simulink model "sdbe_8pac_11"  (R2012b)
settings: Solver=VariableStepDiscrete  SolverMode=SingleTasking  StartTime=0.0  StopTime=10000  RelTol=1e-3
PreLoadFcn:
  | counter_vals
undefined symbols (not defined in the file or in its folder): sfp
libraries: xbsIndex_r4 x9355, casper_library_misc x39, casper_library_delays x27, dspsigops x16, xps_library x10, r2dbe_vdif_lib x4, r2dbe_adc_lib x3, simulink x1
(part 1 of 79)
settings Model: Creator=lvertats  LastModifiedBy=ayoung
settings OptimizationCC: InlineParams=on

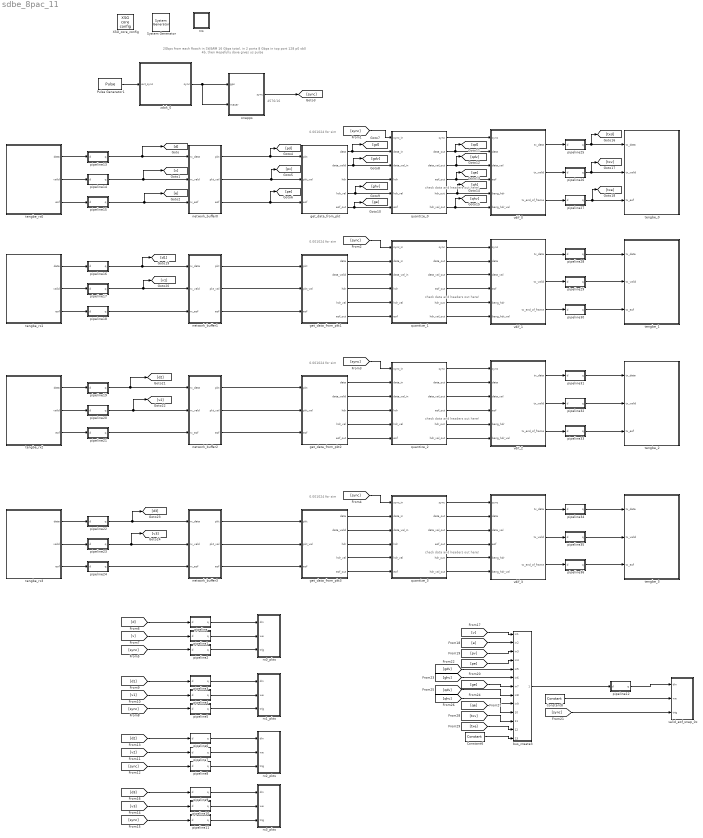
== system sdbe_8pac_11 ==
  note: 0.001024 for sim
  note: 4576/16
  note: check data and headers out here!
  note: 2Gbps from each Roach in SWARM
      | 16 Gbps total, in 2 ports
      | 8 Gbps in top port
      | 128 p0 sb0 4b, then
      |
      | Hopefully dave gives us pulse
  note: 0.001024 for sim
  note: check data and headers out here!
  note: 0.001024 for sim
  note: check data and headers out here!
  note: 0.001024 for sim
  note: check data and headers out here!
  " System Generator" : xbsIndex_r4/ System Generator  Tag=genX  xilinxfamily=virtex6  part=xc6vsx475t  speed=-1  package=ff1759  synthesis_tool=XST  clock_wrapper=Clock Enables  directory=./sdbe_8pac_11/sysgen  proj_type=Project Navigator  Synth_file=XST Defaults  Impl_file=ISE Defaults  testbench=off  simulink_period=1  sysclk_period=3.4965  dcm_input_clock_period=100  incr_netlist=off  trim_vbits=Everywhere in SubSystem  dbl_ovrd=According to Block Masks  core_generation=According to Block Masks  run_coregen=off  deprecated_control=off  eval_field=0  block_type=sysgen
  Constant6 : xbsIndex_r4/Constant  const=0  gui_display_data_type=Fixed-point  arith_type=Unsigned  n_bits=4  bin_pt=0  preci_type=Single  exp_width=8  frac_width=24  explicit_period=on  period=1  equ=P=C  opselect=C  inp2=PCIN>>17  opr=+  inp1=P  carry=CIN  dbl_ovrd=off  block_type=constant
  Constant8 : xbsIndex_r4/Constant  const=1  gui_display_data_type=Boolean  arith_type=Boolean  n_bits=31  bin_pt=0  preci_type=Single  exp_width=8  frac_width=24  explicit_period=on  period=1  equ=P=C  opselect=C  inp2=PCIN>>17  opr=+  inp1=P  carry=CIN  dbl_ovrd=off  block_type=constant
  Pulse Generator1 : DiscretePulseGenerator  Period=1024  PhaseDelay=57
  XSG_core_config : xps_library/XSG core config  Tag=xps:xsg  hw_sys=ROACH2:sx475t  clk_src=adc0_clk  ROACH_clk_src=sys_clk  ROACH2_clk_src=adc0_clk  MKDIG_clk_src=sys_clk  clk_rate=4576/16  sample_period=1  synthesis_tool=XST
  bus_create3 : Subsystem  AncestorBlock=casper_library_flow_control/bus_create  mask(bus_create){inputNum=13}
      mask prompts: inputNum "Number of inputs:"
      mask init:
      | bus_create_init(gcb,...
      |     'inputNum', inputNum);
  get_data_from_pkt : Subsystem
  get_data_from_pkt1 : Subsystem
  get_data_from_pkt2 : Subsystem
  get_data_from_pkt3 : Subsystem
  network_buffer0 : Subsystem  mask{pipe_delay=4}
      mask prompts: pipe_delay "Pipeline delay:"
      mask init:
      | set_param([gcb '/pipe_din'],'latency',pipe_delay)
      | set_param([gcb '/pipe_we'],'latency',pipe_delay)
      | set_param([gcb '/pipe_re'],'latency',pipe_delay)
      | set_param([gcb '/pipe_eof'],'latency',pipe_delay)
  network_buffer1 : Subsystem  mask{pipe_delay=4}
      mask prompts: pipe_delay "Pipeline delay:"
      mask init:
      | set_param([gcb '/pipe_din'],'latency',pipe_delay)
      | set_param([gcb '/pipe_we'],'latency',pipe_delay)
      | set_param([gcb '/pipe_re'],'latency',pipe_delay)
      | set_param([gcb '/pipe_eof'],'latency',pipe_delay)
  network_buffer2 : Subsystem  mask{pipe_delay=4}
      mask prompts: pipe_delay "Pipeline delay:"
      mask init:
      | set_param([gcb '/pipe_din'],'latency',pipe_delay)
      | set_param([gcb '/pipe_we'],'latency',pipe_delay)
      | set_param([gcb '/pipe_re'],'latency',pipe_delay)
      | set_param([gcb '/pipe_eof'],'latency',pipe_delay)
  network_buffer3 : Subsystem  mask{pipe_delay=4}
      mask prompts: pipe_delay "Pipeline delay:"
      mask init:
      | set_param([gcb '/pipe_din'],'latency',pipe_delay)
      | set_param([gcb '/pipe_we'],'latency',pipe_delay)
      | set_param([gcb '/pipe_re'],'latency',pipe_delay)
      | set_param([gcb '/pipe_eof'],'latency',pipe_delay)
  onepps : Subsystem  AncestorBlock=r2dbe_adc_lib/onepps  mask(r2dbe_onepps){clk_rate=4576/16}
      mask prompts: clk_rate "FPGA clock rate (MHz):"
      mask help: Sub-system for 1pps parameters of the R2DBE.
  pipeline : Subsystem  AncestorBlock=casper_library_delays/pipeline  mask(pipeline){latency=16}
      mask help:
      | An explicitly laid-out delay line to avoid mapping to SRL16s
      | for use in pipelining to help achieve timing closure.
      mask init:
      | pipeline_init(gcb,'latency',latency);
      settings: AttributesFormatString=Latency = %<latency>
      mask Display:
      | port_label('input', 1, 'd');
      | port_label('output', 1, 'q');
      | disp(['Z^-', num2str(latency)]);
  pipeline1 : Subsystem  AncestorBlock=casper_library_delays/pipeline  mask(pipeline){latency=16}
      mask help:
      | An explicitly laid-out delay line to avoid mapping to SRL16s
      | for use in pipelining to help achieve timing closure.
      mask init:
      | pipeline_init(gcb,'latency',latency);
      settings: AttributesFormatString=Latency = %<latency>
      mask Display:
      | port_label('input', 1, 'd');
      | port_label('output', 1, 'q');
      | disp(['Z^-', num2str(latency)]);
  pipeline10 : Subsystem  AncestorBlock=casper_library_delays/pipeline  mask(pipeline){latency=16}
      mask help:
      | An explicitly laid-out delay line to avoid mapping to SRL16s
      | for use in pipelining to help achieve timing closure.
      mask init:
      | pipeline_init(gcb,'latency',latency);
      settings: AttributesFormatString=Latency = %<latency>
      mask Display:
      | port_label('input', 1, 'd');
      | port_label('output', 1, 'q');
      | disp(['Z^-', num2str(latency)]);
  pipeline11 : Subsystem  AncestorBlock=casper_library_delays/pipeline  mask(pipeline){latency=16}
      mask help:
      | An explicitly laid-out delay line to avoid mapping to SRL16s
      | for use in pipelining to help achieve timing closure.
      mask init:
      | pipeline_init(gcb,'latency',latency);
      settings: AttributesFormatString=Latency = %<latency>
      mask Display:
      | port_label('input', 1, 'd');
      | port_label('output', 1, 'q');
      | disp(['Z^-', num2str(latency)]);
  pipeline12 : Subsystem  AncestorBlock=casper_library_delays/pipeline  mask(pipeline){latency=16}
      mask help:
      | An explicitly laid-out delay line to avoid mapping to SRL16s
      | for use in pipelining to help achieve timing closure.
      mask init:
      | pipeline_init(gcb,'latency',latency);
      settings: AttributesFormatString=Latency = %<latency>
      mask Display:
      | port_label('input', 1, 'd');
      | port_label('output', 1, 'q');
      | disp(['Z^-', num2str(latency)]);
  pipeline13 : Subsystem  AncestorBlock=casper_library_delays/pipeline  mask(pipeline){latency=4}
      mask help:
      | An explicitly laid-out delay line to avoid mapping to SRL16s
      | for use in pipelining to help achieve timing closure.
      mask init:
      | pipeline_init(gcb,'latency',latency);
      settings: AttributesFormatString=Latency = %<latency>
      mask Display:
      | port_label('input', 1, 'd');
      | port_label('output', 1, 'q');
      | disp(['Z^-', num2str(latency)]);
  pipeline14 : Subsystem  AncestorBlock=casper_library_delays/pipeline  mask(pipeline){latency=4}
      mask help:
      | An explicitly laid-out delay line to avoid mapping to SRL16s
      | for use in pipelining to help achieve timing closure.
      mask init:
      | pipeline_init(gcb,'latency',latency);
      settings: AttributesFormatString=Latency = %<latency>
      mask Display:
      | port_label('input', 1, 'd');
      | port_label('output', 1, 'q');
      | disp(['Z^-', num2str(latency)]);
  pipeline15 : Subsystem  AncestorBlock=casper_library_delays/pipeline  mask(pipeline){latency=4}
      mask help:
      | An explicitly laid-out delay line to avoid mapping to SRL16s
      | for use in pipelining to help achieve timing closure.
      mask init:
      | pipeline_init(gcb,'latency',latency);
      settings: AttributesFormatString=Latency = %<latency>
      mask Display:
      | port_label('input', 1, 'd');
      | port_label('output', 1, 'q');
      | disp(['Z^-', num2str(latency)]);
  pipeline16 : Subsystem  AncestorBlock=casper_library_delays/pipeline  mask(pipeline){latency=4}
      mask help:
      | An explicitly laid-out delay line to avoid mapping to SRL16s
      | for use in pipelining to help achieve timing closure.
      mask init:
      | pipeline_init(gcb,'latency',latency);
      settings: AttributesFormatString=Latency = %<latency>
      mask Display:
      | port_label('input', 1, 'd');
      | port_label('output', 1, 'q');
      | disp(['Z^-', num2str(latency)]);
  pipeline17 : Subsystem  AncestorBlock=casper_library_delays/pipeline  mask(pipeline){latency=4}
      mask help:
      | An explicitly laid-out delay line to avoid mapping to SRL16s
      | for use in pipelining to help achieve timing closure.
      mask init:
      | pipeline_init(gcb,'latency',latency);
      settings: AttributesFormatString=Latency = %<latency>
      mask Display:
      | port_label('input', 1, 'd');
      | port_label('output', 1, 'q');
      | disp(['Z^-', num2str(latency)]);
  pipeline18 : Subsystem  AncestorBlock=casper_library_delays/pipeline  mask(pipeline){latency=4}
      mask help:
      | An explicitly laid-out delay line to avoid mapping to SRL16s
      | for use in pipelining to help achieve timing closure.
      mask init:
      | pipeline_init(gcb,'latency',latency);
      settings: AttributesFormatString=Latency = %<latency>
      mask Display:
      | port_label('input', 1, 'd');
      | port_label('output', 1, 'q');
      | disp(['Z^-', num2str(latency)]);
  pipeline19 : Subsystem  AncestorBlock=casper_library_delays/pipeline  mask(pipeline){latency=4}
      mask help:
      | An explicitly laid-out delay line to avoid mapping to SRL16s
      | for use in pipelining to help achieve timing closure.
      mask init:
      | pipeline_init(gcb,'latency',latency);
      settings: AttributesFormatString=Latency = %<latency>
      mask Display:
      | port_label('input', 1, 'd');
      | port_label('output', 1, 'q');
      | disp(['Z^-', num2str(latency)]);
  pipeline2 : Subsystem  AncestorBlock=casper_library_delays/pipeline  mask(pipeline){latency=16}
      mask help:
      | An explicitly laid-out delay line to avoid mapping to SRL16s
      | for use in pipelining to help achieve timing closure.
      mask init:
      | pipeline_init(gcb,'latency',latency);
      settings: AttributesFormatString=Latency = %<latency>
      mask Display:
      | port_label('input', 1, 'd');
      | port_label('output', 1, 'q');
      | disp(['Z^-', num2str(latency)]);
  pipeline20 : Subsystem  AncestorBlock=casper_library_delays/pipeline  mask(pipeline){latency=4}
      mask help:
      | An explicitly laid-out delay line to avoid mapping to SRL16s
      | for use in pipelining to help achieve timing closure.
      mask init:
      | pipeline_init(gcb,'latency',latency);
      settings: AttributesFormatString=Latency = %<latency>
      mask Display:
      | port_label('input', 1, 'd');
      | port_label('output', 1, 'q');
      | disp(['Z^-', num2str(latency)]);
  pipeline21 : Subsystem  AncestorBlock=casper_library_delays/pipeline  mask(pipeline){latency=4}
      mask help:
      | An explicitly laid-out delay line to avoid mapping to SRL16s
      | for use in pipelining to help achieve timing closure.
      mask init:
      | pipeline_init(gcb,'latency',latency);
      settings: AttributesFormatString=Latency = %<latency>
      mask Display:
      | port_label('input', 1, 'd');
      | port_label('output', 1, 'q');
      | disp(['Z^-', num2str(latency)]);
  pipeline22 : Subsystem  AncestorBlock=casper_library_delays/pipeline  mask(pipeline){latency=4}
      mask help:
      | An explicitly laid-out delay line to avoid mapping to SRL16s
      | for use in pipelining to help achieve timing closure.
      mask init:
      | pipeline_init(gcb,'latency',latency);
      settings: AttributesFormatString=Latency = %<latency>
      mask Display:
      | port_label('input', 1, 'd');
      | port_label('output', 1, 'q');
      | disp(['Z^-', num2str(latency)]);
  pipeline23 : Subsystem  AncestorBlock=casper_library_delays/pipeline  mask(pipeline){latency=4}
      mask help:
      | An explicitly laid-out delay line to avoid mapping to SRL16s
      | for use in pipelining to help achieve timing closure.
      mask init:
      | pipeline_init(gcb,'latency',latency);
      settings: AttributesFormatString=Latency = %<latency>
      mask Display:
      | port_label('input', 1, 'd');
      | port_label('output', 1, 'q');
      | disp(['Z^-', num2str(latency)]);
  pipeline24 : Subsystem  AncestorBlock=casper_library_delays/pipeline  mask(pipeline){latency=4}
      mask help:
      | An explicitly laid-out delay line to avoid mapping to SRL16s
      | for use in pipelining to help achieve timing closure.
      mask init:
      | pipeline_init(gcb,'latency',latency);
      settings: AttributesFormatString=Latency = %<latency>
      mask Display:
      | port_label('input', 1, 'd');
      | port_label('output', 1, 'q');
      | disp(['Z^-', num2str(latency)]);
  pipeline25 : Subsystem  AncestorBlock=casper_library_delays/pipeline  mask(pipeline){latency=4}
      mask help:
      | An explicitly laid-out delay line to avoid mapping to SRL16s
      | for use in pipelining to help achieve timing closure.
      mask init:
      | pipeline_init(gcb,'latency',latency);
      settings: AttributesFormatString=Latency = %<latency>
      mask Display:
      | port_label('input', 1, 'd');
      | port_label('output', 1, 'q');
      | disp(['Z^-', num2str(latency)]);
  pipeline26 : Subsystem  AncestorBlock=casper_library_delays/pipeline  mask(pipeline){latency=4}
      mask help:
      | An explicitly laid-out delay line to avoid mapping to SRL16s
      | for use in pipelining to help achieve timing closure.
      mask init:
      | pipeline_init(gcb,'latency',latency);
      settings: AttributesFormatString=Latency = %<latency>
      mask Display:
      | port_label('input', 1, 'd');
      | port_label('output', 1, 'q');
      | disp(['Z^-', num2str(latency)]);
  pipeline27 : Subsystem  AncestorBlock=casper_library_delays/pipeline  mask(pipeline){latency=4}
      mask help:
      | An explicitly laid-out delay line to avoid mapping to SRL16s
      | for use in pipelining to help achieve timing closure.
      mask init:
      | pipeline_init(gcb,'latency',latency);
      settings: AttributesFormatString=Latency = %<latency>
      mask Display:
      | port_label('input', 1, 'd');
      | port_label('output', 1, 'q');
      | disp(['Z^-', num2str(latency)]);
  pipeline28 : Subsystem  AncestorBlock=casper_library_delays/pipeline  mask(pipeline){latency=4}
      mask help:
      | An explicitly laid-out delay line to avoid mapping to SRL16s
      | for use in pipelining to help achieve timing closure.
      mask init:
      | pipeline_init(gcb,'latency',latency);
      settings: AttributesFormatString=Latency = %<latency>
      mask Display:
      | port_label('input', 1, 'd');
      | port_label('output', 1, 'q');
      | disp(['Z^-', num2str(latency)]);
  pipeline29 : Subsystem  AncestorBlock=casper_library_delays/pipeline  mask(pipeline){latency=4}
      mask help:
      | An explicitly laid-out delay line to avoid mapping to SRL16s
      | for use in pipelining to help achieve timing closure.
      mask init:
      | pipeline_init(gcb,'latency',latency);
      settings: AttributesFormatString=Latency = %<latency>
      mask Display:
      | port_label('input', 1, 'd');
      | port_label('output', 1, 'q');
      | disp(['Z^-', num2str(latency)]);
  pipeline3 : Subsystem  AncestorBlock=casper_library_delays/pipeline  mask(pipeline){latency=16}
      mask help:
      | An explicitly laid-out delay line to avoid mapping to SRL16s
      | for use in pipelining to help achieve timing closure.
      mask init:
      | pipeline_init(gcb,'latency',latency);
      settings: AttributesFormatString=Latency = %<latency>
      mask Display:
      | port_label('input', 1, 'd');
      | port_label('output', 1, 'q');
      | disp(['Z^-', num2str(latency)]);
  pipeline30 : Subsystem  AncestorBlock=casper_library_delays/pipeline  mask(pipeline){latency=4}
      mask help:
      | An explicitly laid-out delay line to avoid mapping to SRL16s
      | for use in pipelining to help achieve timing closure.
      mask init:
      | pipeline_init(gcb,'latency',latency);
      settings: AttributesFormatString=Latency = %<latency>
      mask Display:
      | port_label('input', 1, 'd');
      | port_label('output', 1, 'q');
      | disp(['Z^-', num2str(latency)]);
  pipeline31 : Subsystem  AncestorBlock=casper_library_delays/pipeline  mask(pipeline){latency=4}
      mask help:
      | An explicitly laid-out delay line to avoid mapping to SRL16s
      | for use in pipelining to help achieve timing closure.
      mask init:
      | pipeline_init(gcb,'latency',latency);
      settings: AttributesFormatString=Latency = %<latency>
      mask Display:
      | port_label('input', 1, 'd');
      | port_label('output', 1, 'q');
      | disp(['Z^-', num2str(latency)]);
  pipeline32 : Subsystem  AncestorBlock=casper_library_delays/pipeline  mask(pipeline){latency=4}
      mask help:
      | An explicitly laid-out delay line to avoid mapping to SRL16s
      | for use in pipelining to help achieve timing closure.
      mask init:
      | pipeline_init(gcb,'latency',latency);
      settings: AttributesFormatString=Latency = %<latency>
      mask Display:
      | port_label('input', 1, 'd');
      | port_label('output', 1, 'q');
      | disp(['Z^-', num2str(latency)]);
  pipeline33 : Subsystem  AncestorBlock=casper_library_delays/pipeline  mask(pipeline){latency=4}
      mask help:
      | An explicitly laid-out delay line to avoid mapping to SRL16s
      | for use in pipelining to help achieve timing closure.
      mask init:
      | pipeline_init(gcb,'latency',latency);
      settings: AttributesFormatString=Latency = %<latency>
      mask Display:
      | port_label('input', 1, 'd');
      | port_label('output', 1, 'q');
      | disp(['Z^-', num2str(latency)]);
  pipeline34 : Subsystem  AncestorBlock=casper_library_delays/pipeline  mask(pipeline){latency=4}
      mask help:
      | An explicitly laid-out delay line to avoid mapping to SRL16s
      | for use in pipelining to help achieve timing closure.
      mask init:
      | pipeline_init(gcb,'latency',latency);
      settings: AttributesFormatString=Latency = %<latency>
      mask Display:
      | port_label('input', 1, 'd');
      | port_label('output', 1, 'q');
      | disp(['Z^-', num2str(latency)]);
  pipeline35 : Subsystem  AncestorBlock=casper_library_delays/pipeline  mask(pipeline){latency=4}
      mask help:
      | An explicitly laid-out delay line to avoid mapping to SRL16s
      | for use in pipelining to help achieve timing closure.
      mask init:
      | pipeline_init(gcb,'latency',latency);
      settings: AttributesFormatString=Latency = %<latency>
      mask Display:
      | port_label('input', 1, 'd');
      | port_label('output', 1, 'q');
      | disp(['Z^-', num2str(latency)]);
  pipeline36 : Subsystem  AncestorBlock=casper_library_delays/pipeline  mask(pipeline){latency=4}
      mask help:
      | An explicitly laid-out delay line to avoid mapping to SRL16s
      | for use in pipelining to help achieve timing closure.
      mask init:
      | pipeline_init(gcb,'latency',latency);
      settings: AttributesFormatString=Latency = %<latency>
      mask Display:
      | port_label('input', 1, 'd');
      | port_label('output', 1, 'q');
      | disp(['Z^-', num2str(latency)]);
  pipeline4 : Subsystem  AncestorBlock=casper_library_delays/pipeline  mask(pipeline){latency=16}
      mask help:
      | An explicitly laid-out delay line to avoid mapping to SRL16s
      | for use in pipelining to help achieve timing closure.
      mask init:
      | pipeline_init(gcb,'latency',latency);
      settings: AttributesFormatString=Latency = %<latency>
      mask Display:
      | port_label('input', 1, 'd');
      | port_label('output', 1, 'q');
      | disp(['Z^-', num2str(latency)]);
  pipeline5 : Subsystem  AncestorBlock=casper_library_delays/pipeline  mask(pipeline){latency=16}
      mask help:
      | An explicitly laid-out delay line to avoid mapping to SRL16s
      | for use in pipelining to help achieve timing closure.
      mask init:
      | pipeline_init(gcb,'latency',latency);
      settings: AttributesFormatString=Latency = %<latency>
      mask Display:
      | port_label('input', 1, 'd');
      | port_label('output', 1, 'q');
      | disp(['Z^-', num2str(latency)]);
  pipeline6 : Subsystem  AncestorBlock=casper_library_delays/pipeline  mask(pipeline){latency=16}
      mask help:
      | An explicitly laid-out delay line to avoid mapping to SRL16s
      | for use in pipelining to help achieve timing closure.
      mask init:
      | pipeline_init(gcb,'latency',latency);
      settings: AttributesFormatString=Latency = %<latency>
      mask Display:
      | port_label('input', 1, 'd');
      | port_label('output', 1, 'q');
      | disp(['Z^-', num2str(latency)]);
  pipeline7 : Subsystem  AncestorBlock=casper_library_delays/pipeline  mask(pipeline){latency=16}
      mask help:
      | An explicitly laid-out delay line to avoid mapping to SRL16s
      | for use in pipelining to help achieve timing closure.
      mask init:
      | pipeline_init(gcb,'latency',latency);
      settings: AttributesFormatString=Latency = %<latency>
      mask Display:
      | port_label('input', 1, 'd');
      | port_label('output', 1, 'q');
      | disp(['Z^-', num2str(latency)]);
  pipeline8 : Subsystem  AncestorBlock=casper_library_delays/pipeline  mask(pipeline){latency=16}
      mask help:
      | An explicitly laid-out delay line to avoid mapping to SRL16s
      | for use in pipelining to help achieve timing closure.
      mask init:
      | pipeline_init(gcb,'latency',latency);
      settings: AttributesFormatString=Latency = %<latency>
      mask Display:
      | port_label('input', 1, 'd');
      | port_label('output', 1, 'q');
      | disp(['Z^-', num2str(latency)]);
  pipeline9 : Subsystem  AncestorBlock=casper_library_delays/pipeline  mask(pipeline){latency=16}
      mask help:
      | An explicitly laid-out delay line to avoid mapping to SRL16s
      | for use in pipelining to help achieve timing closure.
      mask init:
      | pipeline_init(gcb,'latency',latency);
      settings: AttributesFormatString=Latency = %<latency>
      mask Display:
      | port_label('input', 1, 'd');
      | port_label('output', 1, 'q');
      | disp(['Z^-', num2str(latency)]);
  quantize_0 : Subsystem  mask(r2dbe_quantize){mult_delay=3, add_delay=2, convert_delay=1, pipeline_delay=1, io_delay=3}
      mask prompts: mult_delay "Multiplier latency:"; add_delay "Adder latency:"; convert_delay "Convert latency:"; pipeline_delay "Output pipeline delay:"; io_delay "I/O delay:"
      mask help: Sub-system for quantization parameters of the R2DBE.
  quantize_1 : Subsystem  mask(r2dbe_quantize){mult_delay=3, add_delay=2, convert_delay=1, pipeline_delay=1, io_delay=3}
      mask prompts: mult_delay "Multiplier latency:"; add_delay "Adder latency:"; convert_delay "Convert latency:"; pipeline_delay "Output pipeline delay:"; io_delay "I/O delay:"
      mask help: Sub-system for quantization parameters of the R2DBE.
  quantize_2 : Subsystem  mask(r2dbe_quantize){mult_delay=3, add_delay=2, convert_delay=1, pipeline_delay=1, io_delay=3}
      mask prompts: mult_delay "Multiplier latency:"; add_delay "Adder latency:"; convert_delay "Convert latency:"; pipeline_delay "Output pipeline delay:"; io_delay "I/O delay:"
      mask help: Sub-system for quantization parameters of the R2DBE.
  quantize_3 : Subsystem  mask(r2dbe_quantize){mult_delay=3, add_delay=2, convert_delay=1, pipeline_delay=1, io_delay=3}
      mask prompts: mult_delay "Multiplier latency:"; add_delay "Adder latency:"; convert_delay "Convert latency:"; pipeline_delay "Output pipeline delay:"; io_delay "I/O delay:"
      mask help: Sub-system for quantization parameters of the R2DBE.
  rcs : Subsystem  AncestorBlock=casper_library_misc/rcs  mask(rcs){app_src=timestamp, lib_src=timestamp, user_val=0}
      mask prompts: app_src "Application revision info to capture"; lib_src "CASPER libraries revision info to capture"; user_val "User specified value"
      mask help:
      | Embeds revision control information for the user design and libraries.
      | On failure to locate specified revision information, falls back to
      | timestamps (current time for libraries).
      | A user specified value is also stored.
      mask init:
      | rcs_init(gcb, ...
      |     'app_src', app_src, ...
      |     'lib_src', lib_src);
      mask TypeOptions app_src: timestamp | git | svn
      mask TypeOptions lib_src: timestamp | git | svn
  rx0_pkts : Subsystem  Tag=casper:snapshot  AncestorBlock=casper_library_scopes/snapshot  mask(snapshot){storage=bram, dram_dimm=1, dram_clock=200, nsamples=14, data_width=64, offset=off, circap=off, value=off, use_dsp48=on}
      mask prompts: storage "Storage medium"; dram_dimm "DRAM dimm"; dram_clock "DRAM clock rate"; nsamples "Number of Samples (2^?)"; data_width "Data width"; offset "Start delay support"; circap "Circular capture support"; value "Extra value capture support"; use_dsp48 "Use DSP48s to implement counters"
      mask help:
      | Standard snap block, but with the following optional extras;
      |  1) Optionally delay the fabric trigger by a user-specified number of valids.
      |  2) Capture continuously after a trigger until a stop pulse is received. Data is captured into BRAM continuously, with old data being overwritten until a stop command is received. Then stop capturing when memory is filled. This enables you to get some data before and some data after the stop pulse. Use the 'tr_en_cnt' register to determine where you are in your vector. 'Addr' register's MSb now indicates 'busy capturing'.
      |  3) Optionally capture a value on an input port to a register at the same time as the first data sample.
      |  4) Implement counters using DSP48Es to save resources.
      mask init:
      | snapshot_init(gcb, ...
      |     'storage', storage, ...
      |     'dram_dimm', dram_dimm, ...
      |     'dram_clock', dram_clock, ...
      |     'nsamples', nsamples, ...
      |     'data_width', data_width, ...
      |     'offset', offset, ...
      |     'circap', circap, ...
      |     'value', value, ...
      |     'use_dsp48', use_dsp48);
      mask TypeOptions storage: bram | dram
      mask Callback storage: snapshot_callback();
      mask TypeOptions dram_dimm: 1 | 2 | 3 | 4
      mask TypeOptions dram_clock: 200 | 250 | 266 | 300 | 333
      mask TypeOptions data_width: 8 | 16 | 32 | 64 | 128
  rx1_pkts : Subsystem  Tag=casper:snapshot  AncestorBlock=casper_library_scopes/snapshot  mask(snapshot){storage=bram, dram_dimm=1, dram_clock=200, nsamples=14, data_width=64, offset=off, circap=off, value=off, use_dsp48=on}
      mask prompts: storage "Storage medium"; dram_dimm "DRAM dimm"; dram_clock "DRAM clock rate"; nsamples "Number of Samples (2^?)"; data_width "Data width"; offset "Start delay support"; circap "Circular capture support"; value "Extra value capture support"; use_dsp48 "Use DSP48s to implement counters"
      mask help:
      | Standard snap block, but with the following optional extras;
      |  1) Optionally delay the fabric trigger by a user-specified number of valids.
      |  2) Capture continuously after a trigger until a stop pulse is received. Data is captured into BRAM continuously, with old data being overwritten until a stop command is received. Then stop capturing when memory is filled. This enables you to get some data before and some data after the stop pulse. Use the 'tr_en_cnt' register to determine where you are in your vector. 'Addr' register's MSb now indicates 'busy capturing'.
      |  3) Optionally capture a value on an input port to a register at the same time as the first data sample.
      |  4) Implement counters using DSP48Es to save resources.
      mask init: same as sdbe_8pac_11/rx0_pkts
      mask TypeOptions storage: bram | dram
      mask Callback storage: snapshot_callback();
      mask TypeOptions dram_dimm: 1 | 2 | 3 | 4
      mask TypeOptions dram_clock: 200 | 250 | 266 | 300 | 333
      mask TypeOptions data_width: 8 | 16 | 32 | 64 | 128
  rx2_pkts : Subsystem  Tag=casper:snapshot  AncestorBlock=casper_library_scopes/snapshot  mask(snapshot){storage=bram, dram_dimm=1, dram_clock=200, nsamples=14, data_width=64, offset=off, circap=off, value=off, use_dsp48=on}
      mask prompts: storage "Storage medium"; dram_dimm "DRAM dimm"; dram_clock "DRAM clock rate"; nsamples "Number of Samples (2^?)"; data_width "Data width"; offset "Start delay support"; circap "Circular capture support"; value "Extra value capture support"; use_dsp48 "Use DSP48s to implement counters"
      mask help:
      | Standard snap block, but with the following optional extras;
      |  1) Optionally delay the fabric trigger by a user-specified number of valids.
      |  2) Capture continuously after a trigger until a stop pulse is received. Data is captured into BRAM continuously, with old data being overwritten until a stop command is received. Then stop capturing when memory is filled. This enables you to get some data before and some data after the stop pulse. Use the 'tr_en_cnt' register to determine where you are in your vector. 'Addr' register's MSb now indicates 'busy capturing'.
      |  3) Optionally capture a value on an input port to a register at the same time as the first data sample.
      |  4) Implement counters using DSP48Es to save resources.
      mask init: same as sdbe_8pac_11/rx0_pkts
      mask TypeOptions storage: bram | dram
      mask Callback storage: snapshot_callback();
      mask TypeOptions dram_dimm: 1 | 2 | 3 | 4
      mask TypeOptions dram_clock: 200 | 250 | 266 | 300 | 333
      mask TypeOptions data_width: 8 | 16 | 32 | 64 | 128
  rx3_pkts : Subsystem  Tag=casper:snapshot  AncestorBlock=casper_library_scopes/snapshot  mask(snapshot){storage=bram, dram_dimm=1, dram_clock=200, nsamples=14, data_width=64, offset=off, circap=off, value=off, use_dsp48=on}
      mask prompts: storage "Storage medium"; dram_dimm "DRAM dimm"; dram_clock "DRAM clock rate"; nsamples "Number of Samples (2^?)"; data_width "Data width"; offset "Start delay support"; circap "Circular capture support"; value "Extra value capture support"; use_dsp48 "Use DSP48s to implement counters"
      mask help:
      | Standard snap block, but with the following optional extras;
      |  1) Optionally delay the fabric trigger by a user-specified number of valids.
      |  2) Capture continuously after a trigger until a stop pulse is received. Data is captured into BRAM continuously, with old data being overwritten until a stop command is received. Then stop capturing when memory is filled. This enables you to get some data before and some data after the stop pulse. Use the 'tr_en_cnt' register to determine where you are in your vector. 'Addr' register's MSb now indicates 'busy capturing'.
      |  3) Optionally capture a value on an input port to a register at the same time as the first data sample.
      |  4) Implement counters using DSP48Es to save resources.
      mask init: same as sdbe_8pac_11/rx0_pkts
      mask TypeOptions storage: bram | dram
      mask Callback storage: snapshot_callback();
      mask TypeOptions dram_dimm: 1 | 2 | 3 | 4
      mask TypeOptions dram_clock: 200 | 250 | 266 | 300 | 333
      mask TypeOptions data_width: 8 | 16 | 32 | 64 | 128
  tengbe_0 : Subsystem  mask(r2dbe_tengbe){slot=0, port=0}
      mask prompts: slot "Card slot:"
      mask help: Sub-system for 10 GbE parameters of the R2DBE.
      mask init:
      | set_param([gcb, '/core'], 'slot', slot);
      | set_param([gcb, '/core'], 'port_r2_sfpp', port);
      mask TypeOptions slot: 0 | 1
      mask TypeOptions port: 0 | 1 | 2 | 3
  tengbe_1 : Subsystem  mask(r2dbe_tengbe){slot=0, port=1}
      mask prompts: slot "Card slot:"
      mask help: Sub-system for 10 GbE parameters of the R2DBE.
      mask init:
      | set_param([gcb, '/core'], 'slot', slot);
      | set_param([gcb, '/core'], 'port_r2_sfpp', port);
      mask TypeOptions slot: 0 | 1
      mask TypeOptions port: 0 | 1 | 2 | 3
  tengbe_2 : Subsystem  mask(r2dbe_tengbe){slot=0, port=2}
      mask prompts: slot "Card slot:"
      mask help: Sub-system for 10 GbE parameters of the R2DBE.
      mask init:
      | set_param([gcb, '/core'], 'slot', slot);
      | set_param([gcb, '/core'], 'port_r2_sfpp', port);
      mask TypeOptions slot: 0 | 1
      mask TypeOptions port: 0 | 1 | 2 | 3
  tengbe_3 : Subsystem  mask(r2dbe_tengbe){slot=0, port=3}
      mask prompts: slot "Card slot:"
      mask help: Sub-system for 10 GbE parameters of the R2DBE.
      mask init:
      | set_param([gcb, '/core'], 'slot', slot);
      | set_param([gcb, '/core'], 'port_r2_sfpp', port);
      mask TypeOptions slot: 0 | 1
      mask TypeOptions port: 0 | 1 | 2 | 3
  tengbe_rx0 : Subsystem  mask(r2dbe_tengbe){slot=1, port=0, pipe_delay=8}
      mask prompts: slot "Card slot:"; pipe_delay "Pipeline delay:"
      mask help: Sub-system for 10 GbE parameters of the R2DBE.
      mask init:
      | set_param([gcb, '/core'], 'slot', slot);
      | set_param([gcb, '/core'], 'port_r2_sfpp', port);
      | set_param([gcb, '/pipe_data'], 'latency', pipe_delay);
      | set_param([gcb, '/pipe_valid'], 'latency', pipe_delay);
      | set_param([gcb, '/pipe_eof'], 'latency', pipe_delay);
      mask TypeOptions slot: 0 | 1
      mask TypeOptions port: 0 | 1 | 2 | 3
  tengbe_rx1 : Subsystem  mask(r2dbe_tengbe){slot=1, port=1, pipe_delay=8}
      mask prompts: slot "Card slot:"; pipe_delay "Pipeline delay:"
      mask help: Sub-system for 10 GbE parameters of the R2DBE.
      mask init: same as sdbe_8pac_11/tengbe_rx0
      mask TypeOptions slot: 0 | 1
      mask TypeOptions port: 0 | 1 | 2 | 3
  tengbe_rx2 : Subsystem  mask(r2dbe_tengbe){slot=1, port=2, pipe_delay=8}
      mask prompts: slot "Card slot:"; pipe_delay "Pipeline delay:"
      mask help: Sub-system for 10 GbE parameters of the R2DBE.
      mask init: same as sdbe_8pac_11/tengbe_rx0
      mask TypeOptions slot: 0 | 1
      mask TypeOptions port: 0 | 1 | 2 | 3
  tengbe_rx3 : Subsystem  mask(r2dbe_tengbe){slot=1, port=3, pipe_delay=8}
      mask prompts: slot "Card slot:"; pipe_delay "Pipeline delay:"
      mask help: Sub-system for 10 GbE parameters of the R2DBE.
      mask init: same as sdbe_8pac_11/tengbe_rx0
      mask TypeOptions slot: 0 | 1
      mask TypeOptions port: 0 | 1 | 2 | 3
  valid_eof_snap_0x : Subsystem  Tag=casper:snapshot  AncestorBlock=casper_library_scopes/snapshot  mask(snapshot){storage=bram, dram_dimm=1, dram_clock=200, nsamples=14, data_width=16, offset=off, circap=off, value=off, use_dsp48=on}
      mask prompts: storage "Storage medium"; dram_dimm "DRAM dimm"; dram_clock "DRAM clock rate"; nsamples "Number of Samples (2^?)"; data_width "Data width"; offset "Start delay support"; circap "Circular capture support"; value "Extra value capture support"; use_dsp48 "Use DSP48s to implement counters"
      mask help:
      | Standard snap block, but with the following optional extras;
      |  1) Optionally delay the fabric trigger by a user-specified number of valids.
      |  2) Capture continuously after a trigger until a stop pulse is received. Data is captured into BRAM continuously, with old data being overwritten until a stop command is received. Then stop capturing when memory is filled. This enables you to get some data before and some data after the stop pulse. Use the 'tr_en_cnt' register to determine where you are in your vector. 'Addr' register's MSb now indicates 'busy capturing'.
      |  3) Optionally capture a value on an input port to a register at the same time as the first data sample.
      |  4) Implement counters using DSP48Es to save resources.
      mask init: same as sdbe_8pac_11/rx0_pkts
      mask TypeOptions storage: bram | dram
      mask Callback storage: snapshot_callback();
      mask TypeOptions dram_dimm: 1 | 2 | 3 | 4
      mask TypeOptions dram_clock: 200 | 250 | 266 | 300 | 333
      mask TypeOptions data_width: 8 | 16 | 32 | 64 | 128
  vdif_0 : Subsystem  mask(r2dbe_vdif){}
      mask help: Sub-system for VDIF parameters of the R2DBE.
  vdif_1 : Subsystem  mask(r2dbe_vdif){}
      mask help: Sub-system for VDIF parameters of the R2DBE.
  vdif_2 : Subsystem  mask(r2dbe_vdif){}
      mask help: Sub-system for VDIF parameters of the R2DBE.
  vdif_3 : Subsystem  mask(r2dbe_vdif){}
      mask help: Sub-system for VDIF parameters of the R2DBE.
  zdok_0 : Subsystem  mask(r2dbe_zdok){zdok=ZDOK 0, nyquist_bw=2288, pipeline_delay=1}
      mask prompts: zdok "ADC board"; nyquist_bw "Nyquist bandwidth (MHz):"; pipeline_delay "Output pipeline delay:"
      mask help: Sub-system for ADC5g parameters of the R2DBE.
      mask init:
      | set_param([gcb, '/adc'], 'adc_brd', zdok);
      mask TypeOptions zdok: ZDOK 0 | ZDOK 1
  wires:
  vdif_0/1(tx_data) -> pipeline25/1(d)
  vdif_0/2(tx_valid) -> pipeline26/1(d)
  vdif_0/3(tx_end_of_frame) -> pipeline27/1(d)
  quantize_0/1(sync) -> vdif_0/1(sync)
  quantize_0/2(data_out) -> vdif_0/2(data), [qd]
  Pulse Generator1/1 -> zdok_0/1(ext_sync)
  zdok_0/1(sync) -> onepps/2(maser), onepps/1(gps)
  onepps/1(sync) -> [sync]
  quantize_0/3(data_val_out) -> vdif_0/3(data_val), [qdv]
  quantize_0/4(eof_out) -> vdif_0/4(eof), [qe]
  quantize_0/5(hdr_out) -> vdif_0/5(beng_hdr), [qh]
  quantize_0/6(hdr_val_out) -> vdif_0/6(beng_hdr_val), [qhv]
  network_buffer0/1(pkt) -> [pd], get_data_from_pkt/1(pkt)
  network_buffer0/2(pkt_val) -> [pv], get_data_from_pkt/2(pkt_val)
  network_buffer0/3(eof) -> [pe], get_data_from_pkt/3(eof)
  get_data_from_pkt/5(eof_out) -> [ge], quantize_0/6(eof)
  get_data_from_pkt/4(hdr_val) -> [ghv], quantize_0/5(hdr_val)
  get_data_from_pkt/3(hdr) -> quantize_0/4(hdr)
  get_data_from_pkt/2(data_valid) -> [gdv], quantize_0/3(data_val_in)
  get_data_from_pkt/1(data) -> [gd], quantize_0/2(data_in)
  [sync] -> quantize_0/1(sync_in)
  quantize_1/1(sync) -> vdif_1/1(sync)
  quantize_1/2(data_out) -> vdif_1/2(data)
  quantize_1/3(data_val_out) -> vdif_1/3(data_val)
  quantize_1/4(eof_out) -> vdif_1/4(eof)
  quantize_1/5(hdr_out) -> vdif_1/5(beng_hdr)
  quantize_1/6(hdr_val_out) -> vdif_1/6(beng_hdr_val)
  network_buffer1/1(pkt) -> get_data_from_pkt1/1(pkt)
  network_buffer1/2(pkt_val) -> get_data_from_pkt1/2(pkt_val)
  network_buffer1/3(eof) -> get_data_from_pkt1/3(eof)
  get_data_from_pkt1/5(eof_out) -> quantize_1/6(eof)
  get_data_from_pkt1/4(hdr_val) -> quantize_1/5(hdr_val)
  get_data_from_pkt1/3(hdr) -> quantize_1/4(hdr)
  get_data_from_pkt1/2(data_valid) -> quantize_1/3(data_val_in)
  get_data_from_pkt1/1(data) -> quantize_1/2(data_in)
  [sync] -> quantize_1/1(sync_in)
  quantize_2/1(sync) -> vdif_2/1(sync)
  quantize_2/2(data_out) -> vdif_2/2(data)
  quantize_2/3(data_val_out) -> vdif_2/3(data_val)
  quantize_2/4(eof_out) -> vdif_2/4(eof)
  quantize_2/5(hdr_out) -> vdif_2/5(beng_hdr)
  quantize_2/6(hdr_val_out) -> vdif_2/6(beng_hdr_val)
  network_buffer2/1(pkt) -> get_data_from_pkt2/1(pkt)
  network_buffer2/2(pkt_val) -> get_data_from_pkt2/2(pkt_val)
  network_buffer2/3(eof) -> get_data_from_pkt2/3(eof)
  get_data_from_pkt2/5(eof_out) -> quantize_2/6(eof)
  get_data_from_pkt2/4(hdr_val) -> quantize_2/5(hdr_val)
  get_data_from_pkt2/3(hdr) -> quantize_2/4(hdr)
  get_data_from_pkt2/2(data_valid) -> quantize_2/3(data_val_in)
  get_data_from_pkt2/1(data) -> quantize_2/2(data_in)
  [sync] -> quantize_2/1(sync_in)
  quantize_3/1(sync) -> vdif_3/1(sync)
  quantize_3/2(data_out) -> vdif_3/2(data)
  quantize_3/3(data_val_out) -> vdif_3/3(data_val)
  quantize_3/4(eof_out) -> vdif_3/4(eof)
  quantize_3/5(hdr_out) -> vdif_3/5(beng_hdr)
  quantize_3/6(hdr_val_out) -> vdif_3/6(beng_hdr_val)
  network_buffer3/1(pkt) -> get_data_from_pkt3/1(pkt)
  network_buffer3/2(pkt_val) -> get_data_from_pkt3/2(pkt_val)
  network_buffer3/3(eof) -> get_data_from_pkt3/3(eof)
  get_data_from_pkt3/5(eof_out) -> quantize_3/6(eof)
  get_data_from_pkt3/4(hdr_val) -> quantize_3/5(hdr_val)
  get_data_from_pkt3/3(hdr) -> quantize_3/4(hdr)
  get_data_from_pkt3/2(data_valid) -> quantize_3/3(data_val_in)
  get_data_from_pkt3/1(data) -> quantize_3/2(data_in)
  [sync] -> quantize_3/1(sync_in)
  Constant8/1 -> valid_eof_snap_0x/2(we)
  [sync] -> valid_eof_snap_0x/3(trig)
  [e] -> bus_create3/2(in2)
  [v] -> bus_create3/1(in1)
  [pv] -> bus_create3/3(in3)
  [pe] -> bus_create3/4(in4)
  [gdv] -> bus_create3/5(in5)
  [ghv] -> bus_create3/6(in6)
  [qdv] -> bus_create3/8(in8)
  [qhv] -> bus_create3/9(in9)
  [ge] -> bus_create3/7(in7)
  [qe] -> bus_create3/10(in10)
  [txv] -> bus_create3/11(in11)
  [txe] -> bus_create3/12(in12)
  Constant6/1 -> bus_create3/13(in13)
  pipeline/1(q) -> rx0_pkts/1(din)
  pipeline1/1(q) -> rx0_pkts/2(we)
  pipeline2/1(q) -> rx0_pkts/3(trig)
  [d] -> pipeline/1(d)
  [v] -> pipeline1/1(d)
  [sync] -> pipeline2/1(d)
  pipeline3/1(q) -> rx1_pkts/1(din)
  pipeline4/1(q) -> rx1_pkts/2(we)
  pipeline5/1(q) -> rx1_pkts/3(trig)
  [d1] -> pipeline3/1(d)
  [v1] -> pipeline4/1(d)
  [sync] -> pipeline5/1(d)
  pipeline6/1(q) -> rx2_pkts/1(din)
  pipeline7/1(q) -> rx2_pkts/2(we)
  pipeline8/1(q) -> rx2_pkts/3(trig)
  [d2] -> pipeline6/1(d)
  [v2] -> pipeline7/1(d)
  [sync] -> pipeline8/1(d)
  pipeline9/1(q) -> rx3_pkts/1(din)
  pipeline10/1(q) -> rx3_pkts/2(we)
  pipeline11/1(q) -> rx3_pkts/3(trig)
  [d3] -> pipeline9/1(d)
  [v3] -> pipeline10/1(d)
  [sync] -> pipeline11/1(d)
  pipeline12/1(q) -> valid_eof_snap_0x/1(din)
  bus_create3/1(bus_out) -> pipeline12/1(d)
  pipeline15/1(q) -> [e], network_buffer0/3(rx_eof)
  pipeline13/1(q) -> [d], network_buffer0/1(rx_data)
  tengbe_rx0/1(data) -> pipeline13/1(d)
  tengbe_rx0/2(valid) -> pipeline14/1(d)
  tengbe_rx0/3(eof) -> pipeline15/1(d)
  pipeline14/1(q) -> [v], network_buffer0/2(rx_vald)
  pipeline18/1(q) -> network_buffer1/3(rx_eof)
  pipeline16/1(q) -> [d1], network_buffer1/1(rx_data)
  tengbe_rx1/1(data) -> pipeline16/1(d)
  tengbe_rx1/2(valid) -> pipeline17/1(d)
  tengbe_rx1/3(eof) -> pipeline18/1(d)
  pipeline17/1(q) -> [v1], network_buffer1/2(rx_vald)
  tengbe_rx2/1(data) -> pipeline19/1(d)
  tengbe_rx2/2(valid) -> pipeline20/1(d)
  tengbe_rx2/3(eof) -> pipeline21/1(d)
  pipeline19/1(q) -> [d2], network_buffer2/1(rx_data)
  pipeline20/1(q) -> [v2], network_buffer2/2(rx_vald)
  pipeline21/1(q) -> network_buffer2/3(rx_eof)
  tengbe_rx3/1(data) -> pipeline22/1(d)
  tengbe_rx3/2(valid) -> pipeline23/1(d)
  tengbe_rx3/3(eof) -> pipeline24/1(d)
  pipeline22/1(q) -> [d3], network_buffer3/1(rx_data)
  pipeline23/1(q) -> [v3], network_buffer3/2(rx_vald)
  pipeline24/1(q) -> network_buffer3/3(rx_eof)
  pipeline25/1(q) -> [txd], tengbe_0/1(tx_data)
  pipeline26/1(q) -> [txv], tengbe_0/2(tx_valid)
  pipeline27/1(q) -> [txe], tengbe_0/3(tx_eof)
  vdif_1/3(tx_end_of_frame) -> pipeline30/1(d)
  pipeline30/1(q) -> tengbe_1/3(tx_eof)
  pipeline29/1(q) -> tengbe_1/2(tx_valid)
  vdif_1/2(tx_valid) -> pipeline29/1(d)
  vdif_1/1(tx_data) -> pipeline28/1(d)
  pipeline28/1(q) -> tengbe_1/1(tx_data)
  vdif_2/3(tx_end_of_frame) -> pipeline33/1(d)
  pipeline33/1(q) -> tengbe_2/3(tx_eof)
  pipeline32/1(q) -> tengbe_2/2(tx_valid)
  vdif_2/2(tx_valid) -> pipeline32/1(d)
  vdif_2/1(tx_data) -> pipeline31/1(d)
  pipeline31/1(q) -> tengbe_2/1(tx_data)
  vdif_3/1(tx_data) -> pipeline34/1(d)
  pipeline34/1(q) -> tengbe_3/1(tx_data)
  vdif_3/2(tx_valid) -> pipeline35/1(d)
  pipeline35/1(q) -> tengbe_3/2(tx_valid)
  vdif_3/3(tx_end_of_frame) -> pipeline36/1(d)
  pipeline36/1(q) -> tengbe_3/3(tx_eof)

== system sdbe_8pac_11/bus_create3 ==
  in1 : Inport
  in2 : Inport  Port=2
  in3 : Inport  Port=3
  in4 : Inport  Port=4
  in5 : Inport  Port=5
  in6 : Inport  Port=6
  in7 : Inport  Port=7
  in8 : Inport  Port=8
  in9 : Inport  Port=9
  in10 : Inport  Port=10
  in11 : Inport  Port=11
  in12 : Inport  Port=12
  in13 : Inport  Port=13
  concatenate : xbsIndex_r4/Concat  num_inputs=13  dbl_ovrd=off  block_type=concat
  reinterpret{1..13} (13 alike) : xbsIndex_r4/Reinterpret  force_arith_type=on  arith_type=Unsigned  force_bin_pt=on  bin_pt=0  block_type=reinterpret
      reinterpret1 settings: infoedit="Changes signal type without altering the binary representation.   You can changed the signal between signed and unsigned, and relocate the binary point.<br><br>Hardware notes: In hardware this block costs nothing.<br><br>Example:  Suppose the input is 6 bits wide, signed, with 2 fractional bits, and the output is forced to unsigned with 0 fractional bits.  Then an input of -2.0 (1110.00 in binary 2's complement) becomes an output of 56 (111000 in binary)."
      reinterpret2 settings: infoedit="Changes signal type without altering the binary representation.   You can changed the signal between signed and unsigned, and relocate the binary point.<br><br>Hardware notes: In hardware this block costs nothing.<br><br>Example:  Suppose the input is 6 bits wide, signed, with 2 fractional bits, and the output is forced to unsigned with 0 fractional bits.  Then an input of -2.0 (1110.00 in binary 2's complement) becomes an output of 56 (111000 in binary)."
  bus_out : Outport
  wires:
  concatenate/1 -> bus_out/1
  in1/1 -> reinterpret1/1
  reinterpret1/1 -> concatenate/1
  in2/1 -> reinterpret2/1
  reinterpret2/1 -> concatenate/2
  in3/1 -> reinterpret3/1
  reinterpret3/1 -> concatenate/3
  in4/1 -> reinterpret4/1
  reinterpret4/1 -> concatenate/4
  in5/1 -> reinterpret5/1
  reinterpret5/1 -> concatenate/5
  in6/1 -> reinterpret6/1
  reinterpret6/1 -> concatenate/6
  in7/1 -> reinterpret7/1
  reinterpret7/1 -> concatenate/7
  in8/1 -> reinterpret8/1
  reinterpret8/1 -> concatenate/8
  in9/1 -> reinterpret9/1
  reinterpret9/1 -> concatenate/9
  in10/1 -> reinterpret10/1
  reinterpret10/1 -> concatenate/10
  in11/1 -> reinterpret11/1
  reinterpret11/1 -> concatenate/11
  in12/1 -> reinterpret12/1
  reinterpret12/1 -> concatenate/12
  in13/1 -> reinterpret13/1
  reinterpret13/1 -> concatenate/13
